simulink model "BEML_EMU_TestBench_6Car"  (R2019b)
settings: Solver=VariableStepAuto  StartTime=0.0  StopTime=inf  RelTol=1e-3
PreLoadFcn:
  | set_up_test_modelCB_6Car;
undefined symbols (not defined in the file): Common, IOControls, MaxVehicles, MotionBaseControllerInput, VehicleInputs, VehicleType, Z_CfgVehBus
libraries: TestBenchLib x583, simulink x6
(part 1 of 3)
settings Model: EnablePacing=on  Creator=bnadpurohit  LastModifiedBy=hinganes
settings DebuggingCC: FrameProcessingCompatibilityMsg=warning

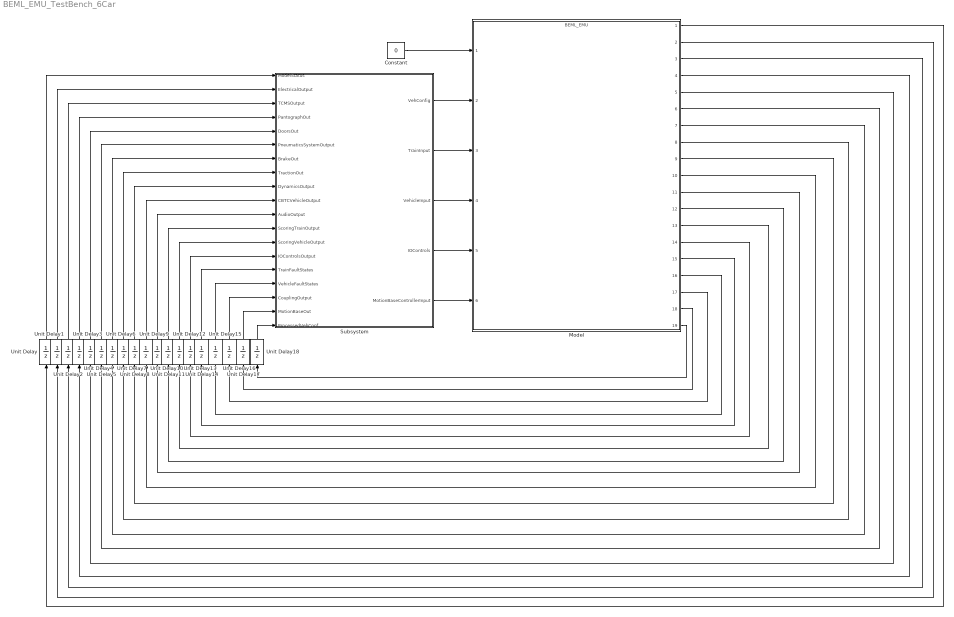
== system BEML_EMU_TestBench_6Car ==
  Constant : Constant  Value=0  OutDataTypeStr=Bus: BD_CommonTrain_SimulatorData
  Model : ModelReference  ModelNameDialog=BEML_EMU.slx  ParameterArgumentNames=PRM_SimIntegration  ParameterArgumentValues=Z_SimIntegrationPrm  UsingDefaultArgumentValue=0  SimulationMode=Normal  ModelReferenceVersion=1.1242
  Subsystem : Subsystem  TreatAsAtomicUnit=on  SystemSampleTime=0.05
  Unit Delay{,1..18} (19 alike) : UnitDelay  SampleTime=-1  HasFrameUpgradeWarning=on
  wires:
  Model/13 -> Unit Delay12/1
  Model/18 -> Unit Delay17/1
  Unit Delay17/1 -> Subsystem/18(MotionBaseOut)
  Model/1 -> Unit Delay/1
  Model/5 -> Unit Delay4/1
  Subsystem/1(VehConfig) -> Model/2
  Model/10 -> Unit Delay9/1
  Model/6 -> Unit Delay5/1
  Unit Delay18/1 -> Subsystem/19(ProcessedVehConf)
  Model/19 -> Unit Delay18/1
  Model/15 -> Unit Delay14/1
  Unit Delay10/1 -> Subsystem/11(AudioOutput)
  Unit Delay6/1 -> Subsystem/7(BrakeOut)
  Subsystem/2(TrainInput) -> Model/3
  Subsystem/5(MotionBaseControllerInput) -> Model/6
  Unit Delay12/1 -> Subsystem/13(ScoringVehicleOutput)
  Unit Delay14/1 -> Subsystem/15(TrainFaultStates)
  Unit Delay2/1 -> Subsystem/3(TCMSOutput)
  Subsystem/3(VehicleInput) -> Model/4
  Unit Delay8/1 -> Subsystem/9(DynamicsOutput)
  Unit Delay11/1 -> Subsystem/12(ScoringTrainOutput)
  Model/4 -> Unit Delay3/1
  Model/2 -> Unit Delay1/1
  Unit Delay1/1 -> Subsystem/2(ElectricalOutput)
  Constant/1 -> Model/1
  Model/12 -> Unit Delay11/1
  Unit Delay4/1 -> Subsystem/5(DoorsOut)
  Unit Delay/1 -> Subsystem/1(ModelStatus)
  Unit Delay15/1 -> Subsystem/16(VehicleFaultStates)
  Model/3 -> Unit Delay2/1
  Unit Delay5/1 -> Subsystem/6(PneumaticsSystemOutput)
  Model/9 -> Unit Delay8/1
  Model/11 -> Unit Delay10/1
  Model/16 -> Unit Delay15/1
  Unit Delay3/1 -> Subsystem/4(PantographOut)
  Model/7 -> Unit Delay6/1
  Model/8 -> Unit Delay7/1
  Subsystem/4(IOControls) -> Model/5
  Unit Delay9/1 -> Subsystem/10(CBTCVehicleOutput)
  Unit Delay13/1 -> Subsystem/14(IOControlsOutput)
  Unit Delay7/1 -> Subsystem/8(TractionOut)
  Model/17 -> Unit Delay16/1
  Unit Delay16/1 -> Subsystem/17(CouplingOutput)
  Model/14 -> Unit Delay13/1

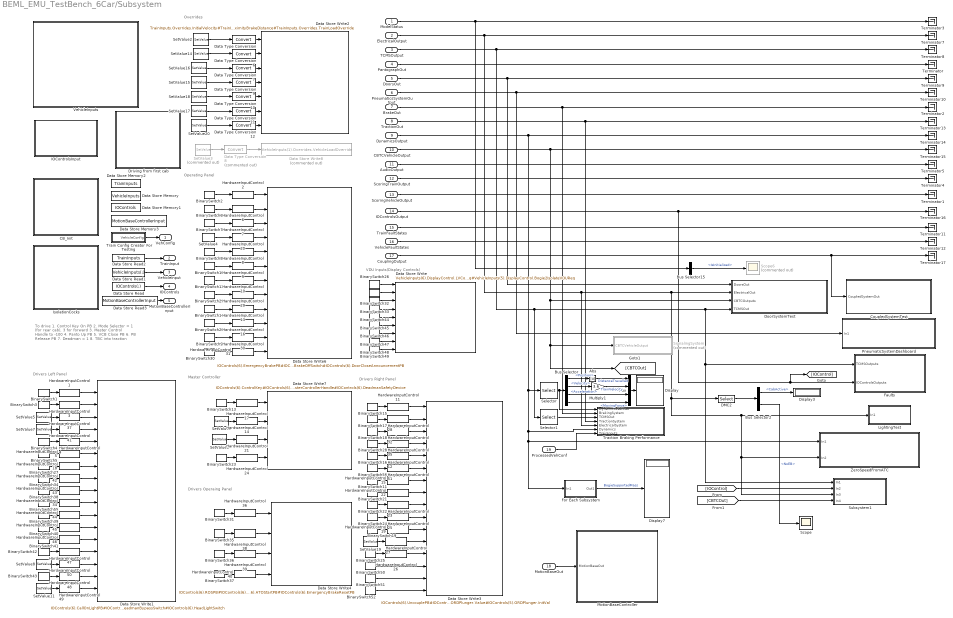
== system BEML_EMU_TestBench_6Car/Subsystem ==
  note: Operating Panel
  note: To drive
      | 1. Control Key On PB
      | 2. Mode Selector = 1 (for rear cab), 3 for forward
      | 3. Master Control Handle to -100
      | 4. Panto Up PB
      | 5. VCB Close PB
      | 6. PB Release PB
      | 7. Deadman = 1
      | 8. TBC into traction
  note: Drivers Operaing Panel
  note: Master Controller
  note: Drivers Right Panel
  note: Drivers Left Panel
  note: VDU Inputs(Display Controls)
  note: Overrides
  ModelStatus : Inport
  ElectricalOutput : Inport  Port=2
  TCMSOutput : Inport  Port=3
  PantographOut : Inport  Port=4
  DoorsOut : Inport  Port=5
  PneumaticsSystemOutput : Inport  Port=6
  BrakeOut : Inport  Port=7
  TractionOut : Inport  Port=8
  DynamicsOutput : Inport  Port=9
  CBTCVehicleOutput : Inport  Port=10
  AudioOutput : Inport  Port=11
  ScoringTrainOutput : Inport  Port=12
  ScoringVehicleOutput : Inport  Port=13
  IOControlsOutput : Inport  Port=14
  TrainFaultStates : Inport  Port=15
  VehicleFaultStates : Inport  Port=16
  CouplingOutput : Inport  Port=17
  MotionBaseOut : Inport  Port=18
  ProcessedVehConf : Inport  Port=19
  Abs : Abs
  BinarySwitch{1..22,24..49,51..52,55..56} (52 alike) : TestBenchLib/BinarySwitch  value=0  init_value=0  block_colour=[0 1 0]  WorkspaceVarName=0
      settings: SourceProductName=Sydac Utilities
  BinarySwitch23 : TestBenchLib/BinarySwitch  value=1  init_value=1  block_colour=[0 1 0]  WorkspaceVarName=0
      settings: SourceProductName=Sydac Utilities
  BinarySwitch50 : TestBenchLib/BinarySwitch  value=1  init_value=1  block_colour=[0 1 0]  WorkspaceVarName=0
      settings: SourceProductName=Sydac Utilities
  Bus Selector : BusSelector  OutputSignals=Inertia.Position,Inertia.Velocity,Inertia.Acceleration,Inertia.MovingForce
  Bus Selector15 : BusSelector  OutputSignals=IsInitialized
  Bus Selector2 : BusSelector  OutputSignals=TCMS.CabActive,TCMS.NoEB
  CB_Init : Subsystem
  CoupledSystemTest : Subsystem
  DMC2 : Selector  InputPortWidth=MaxVehicles  IndexOptions=Index vector (dialog)  Indices=6  OutputSizes=1
  Data Store Memory : DataStoreMemory  DataStoreName=VehicleInputs  ReadBeforeWriteMsg=warning  WriteAfterWriteMsg=warning  WriteAfterReadMsg=warning  ShowAdditionalParam=off  OutDataTypeStr=Bus: BD_SimIntegration_In_Vehicle  Dimensions=MaxVehicles
  Data Store Memory1 : DataStoreMemory  Priority=1  DataStoreName=IOControls  ReadBeforeWriteMsg=warning  WriteAfterWriteMsg=warning  WriteAfterReadMsg=warning  ShowAdditionalParam=off  OutDataTypeStr=Bus: BD_IOControls_In_Vehicle  Dimensions=MaxVehicles
  Data Store Memory2 : DataStoreMemory  DataStoreName=TrainInputs  ReadBeforeWriteMsg=warning  WriteAfterWriteMsg=warning  WriteAfterReadMsg=warning  ShowAdditionalParam=off  OutDataTypeStr=Bus: BD_SimIntegration_In_Train
  Data Store Memory3 : DataStoreMemory  Priority=1  DataStoreName=MotionBaseControllerInput  ReadBeforeWriteMsg=warning  WriteAfterWriteMsg=warning  WriteAfterReadMsg=warning  ShowAdditionalParam=off  OutDataTypeStr=Bus: BD_SimIntegration_In_Vehicle_MotionBaseController  Dimensions=MaxVehicles
  Data Store Read : DataStoreRead  Priority=2  DataStoreName=IOControls  DataStoreElements=IOControls(:)
  Data Store Read1 : DataStoreRead  Priority=2  DataStoreName=VehicleInputs  DataStoreElements=VehicleInputs(:)
  Data Store Read2 : DataStoreRead  Priority=2  DataStoreName=TrainInputs  DataStoreElements=TrainInputs
  Data Store Read3 : DataStoreRead  Priority=2  DataStoreName=MotionBaseControllerInput  DataStoreElements=MotionBaseControllerInput
  Data Store Write : DataStoreWrite  DataStoreName=VehicleInputs  DataStoreElements=VehicleInputs(6).DisplayControl.LVCommandPOPB#VehicleInputs(3).DisplayControl.LVIsolateBCG1#VehicleInputs(3).DisplayControl.LVIsolateBCG2#VehicleInputs(4).DisplayControl.LVIsolateBCG1#VehicleInputs(4).DisplayControl.LVIsolateBCG2#VehicleInputs(6).DisplayControl.Bogie1IsolateVDUReq#VehicleInputs(6).DisplayControl.Bogie2IsolateVDUReq#VehicleInputs(5).DisplayControl.Bogie1IsolateVDUReq#VehicleInputs(5).DisplayControl.Bogie2IsolateVDUReq
  Data Store Write1 : DataStoreWrite  Priority=1  DataStoreName=IOControls  DataStoreElements=IOControls(6).CallOnLightPB#IOControls(6).VCBOpenPB#IOControls(6).WiperSelectionSwitch#IOControls(6).WiperControlSwitch#IOControls(6).LIMPHomePB#IOControls(6).PowerOffPB#IOControls(6).PantoDownPB#IOControls(6).VCBClosePB#IOControls(6).LeftDoorOpenPBOperatingPanel2#IOControls(6).LeftDoorOpenPB1OperatingPanel2#IOControls(6).LeftDoorClosePBOperatingPanel2#IOControls(6).PantoUpPB#IOControls(6).SafetyCutoutSS#IOControls(6).BrakeLoopCutoutSS#IOControls(6).PantoSelector#IOControls(6).DeadmanBypassSwitch#IOControls(6).HeadLightSwitch
  Data Store Write2 : DataStoreWrite  Priority=1  DataStoreName=TrainInputs  DataStoreElements=TrainInputs.Overrides.InitialVelocity#TrainInputs.CBTCTuning.ATOTractionP#TrainInputs.CBTCTuning.ATOTractionI#TrainInputs.CBTCTuning.ATOBrakeP#TrainInputs.CBTCTuning.ATOBrakeI#TrainInputs.CBTCTuning.ATOProximityBrakeDistance#TrainInputs.Overrides.TrainLoadOverride
  Data Store Write3 : DataStoreWrite  Priority=1  DataStoreName=IOControls  DataStoreElements=IOControls(6).UncouplePB#IOControls(6).FlasherLightPB#IOControls(6).FloodLightPB#IOControls(6).BatteryResetPB#IOControls(6).RightDoorOpenPBOperatingPanel5#IOControls(6).RightDoorOpenPB1OperatingPanel5#IOControls(6).RightDoorClosePBOperatingPanel5#IOControls(6).DoorProvenLoopOutputSwitch#IOControls(6).LampTestPB#IOControls(6).WFLTestPB#IOControls(6).EmergencyStopPB#IOControls(6).HoldDoorCloseBypassSS#IOControls(6).EmergencyBrakePBBypassSS#IOControls(5).ORDPlunger.Mode#IOControls(5).ORDPlunger.Value#IOControls(5).ORDPlunger.InitVal
  Data Store Write4 : DataStoreWrite  Priority=1  DataStoreName=IOControls  DataStoreElements=IOControls(6).ROSPB#IOControls(6).UTOPB#IOControls(6).ATOStartPB#IOControls(6).EmergencyBrakeResetPB
  Data Store Write6 : DataStoreWrite  Priority=1  DataStoreName=IOControls  DataStoreElements=IOControls(6).EmergencyBrakePB#IOControls(6).HornPB#IOControls(6).CabConsoleLightPB#IOControls(6).DoorProvenLoopCutoutPB#IOControls(6).LeftDoorClosePBOperatingPanel1#IOControls(6).RightDoorClosePBOperatingPanel1#IOControls(6).LeftDoorOpenPBOperatingPanel1#IOControls(6).RightDoorOpenPBOperatingPanel1#IOControls(6).CabMainLightPB#IOControls(6).ParkingBrakeOnSwitch#IOControls(6).ParkingBrakeOffSwitch#IOControls(6).DoorCloseAnnouncementPB
  Data Store Write7 : DataStoreWrite  Priority=1  DataStoreName=IOControls  DataStoreElements=IOControls(6).ControlKey#IOControls(6).ModeSelector#IOControls(6).MasterControllerHandle#IOControls(6).DeadmanSafetyDevice
  Data Store Write8 : DataStoreWrite  Priority=1  Commented=on  DataStoreName=VehicleInputs  DataStoreElements=VehicleInputs(1).Overrides.VehicleLoadOverride
  Data Type Conversion{,6..7,9..12} (7 alike) : DataTypeConversion
  Data Type Conversion8 : DataTypeConversion  Commented=on
  Display : Display
  Display3 : Display
  Display7 : Display
  DoorSystemTest : Subsystem
  Driving from first cab : Subsystem
  Faults : Subsystem
  For Each Subsystem : Subsystem  TreatAsAtomicUnit=on
  HardwareInputControl{1..32,34..51} (50 alike) : TestBenchLib/HardwareInputControl
      settings: SourceProductName=Sydac Utilities
  IOControlsInput : Subsystem
  IsolationCocks : Subsystem
  LightingTest : Subsystem
  MotionBaseController : Subsystem
  Multiply1 : Gain  Gain=3.6
  Mux : Mux
  PneumaticSystemDashboard : Subsystem
  Scope : Scope
  Scope6 : Scope  Commented=on
  Selector : Selector  InputPortWidth=MaxVehicles  IndexOptions=Index vector (dialog)  Indices=6  OutputSizes=1
  Selector1 : Selector  InputPortWidth=MaxVehicles  IndexOptions=Index vector (dialog)  Indices=6  OutputSizes=1
  SetValue1 : TestBenchLib/SetValue  value=-100  init_value=-100  WorkspaceVarName=0
      settings: SourceProductName=Sydac Utilities
  SetValue{2,4..8,11,19..20} (9 alike) : TestBenchLib/SetValue  value=0  init_value=0  WorkspaceVarName=0
      settings: SourceProductName=Sydac Utilities
  SetValue14 : TestBenchLib/SetValue  value=50  init_value=50  WorkspaceVarName=0
      settings: SourceProductName=Sydac Utilities
  SetValue15 : TestBenchLib/SetValue  value=100  init_value=100  WorkspaceVarName=0
      settings: SourceProductName=Sydac Utilities
  SetValue16 : TestBenchLib/SetValue  value=2  init_value=2  WorkspaceVarName=0
      settings: SourceProductName=Sydac Utilities
  SetValue17 : TestBenchLib/SetValue  value=0.5  init_value=0.5  WorkspaceVarName=0
      settings: SourceProductName=Sydac Utilities
  SetValue18 : TestBenchLib/SetValue  value=5  init_value=5  WorkspaceVarName=0
      settings: SourceProductName=Sydac Utilities
  SetValue3 : TestBenchLib/SetValue  Commented=on  value=0  init_value=0  WorkspaceVarName=0
      settings: SourceProductName=Sydac Utilities
  SignalingSystem : Subsystem  Commented=on
  Subsystem1 : Subsystem
  Terminator{,1..5,7..17} (17 alike) : Terminator
  Traction Braking Performance : Subsystem
  Train Config Creator For Testing : Subsystem
  VehicleInputs : Subsystem
  ZeroSpeedFromATC : Subsystem
  VehConfig : Outport  VectorParamsAs1DForOutWhenUnconnected=off
  TrainInput : Outport  Port=2  VectorParamsAs1DForOutWhenUnconnected=off
  VehicleInput : Outport  Port=3  VectorParamsAs1DForOutWhenUnconnected=off
  IOControls : Outport  Port=4  VectorParamsAs1DForOutWhenUnconnected=off
  MotionBaseControllerInput : Outport  Port=5  VectorParamsAs1DForOutWhenUnconnected=off
  wires:
  BinarySwitch32/1 -> Data Store Write/2
  HardwareInputControl44/1 -> Data Store Write1/11
  BinarySwitch29/1 -> HardwareInputControl29/1
  Selector1/1 -> Traction Braking Performance/3(TCMSOut)
  SetValue4/1 -> HardwareInputControl20/1
  BinarySwitch1/1 -> HardwareInputControl1/1
  SetValue2/1 -> Data Type Conversion/1
  BinarySwitch17/1 -> HardwareInputControl28/1
  BinarySwitch33/1 -> Data Store Write/3
  BinarySwitch13/1 -> HardwareInputControl17/1
  Bus Selector15/1 -> Scope6/1  "<IsInitialized>"
  BinarySwitch56/1 -> HardwareInputControl51/1
  SetValue17/1 -> Data Type Conversion11/1
  Data Type Conversion6/1 -> Data Store Write2/2
  BinarySwitch45/1 -> Data Store Write/5
  Data Type Conversion/1 -> Data Store Write2/1
  SetValue18/1 -> Data Type Conversion10/1
  Data Type Conversion8/1 -> Data Store Write8/1
  HardwareInputControl42/1 -> Data Store Write1/8
  SetValue16/1 -> Data Type Conversion7/1
  Data Type Conversion7/1 -> Data Store Write2/3
  SetValue15/1 -> Data Type Conversion9/1
  HardwareInputControl25/1 -> Data Store Write3/10
  BinarySwitch30/1 -> HardwareInputControl31/1
  Data Type Conversion9/1 -> Data Store Write2/4
  Data Type Conversion10/1 -> Data Store Write2/5
  BinarySwitch12/1 -> HardwareInputControl10/1
  Bus Selector/4 -> Mux/4  "<MovingForce>"
  SetValue5/1 -> HardwareInputControl37/1
  BinarySwitch49/1 -> Data Store Write/9
  BinarySwitch44/1 -> Data Store Write/4
  DMC2/1 -> Bus Selector2/1
  TrainFaultStates/1 -> Terminator11/1
  BinarySwitch47/1 -> Data Store Write/7
  For Each Subsystem/1(Out1) -> Display7/1  "BogieSupportedMass"
  BinarySwitch26/1 -> Data Store Write/1
  HardwareInputControl16/1 -> Data Store Write6/10
  Data Store Read2/1 -> TrainInput/1
  BinarySwitch48/1 -> Data Store Write/8
  HardwareInputControl45/1 -> Data Store Write1/12
  SetValue1/1 -> HardwareInputControl21/1
  Data Type Conversion11/1 -> Data Store Write2/6
  BinarySwitch7/1 -> HardwareInputControl7/1
  SetValue14/1 -> Data Type Conversion6/1
  Mux/1 -> Display/1
  CouplingOutput/1 -> Terminator17/1, CoupledSystemTest/1(CoupledSystemOut)
  Data Type Conversion12/1 -> Data Store Write2/7
  ElectricalOutput/1 -> Terminator7/1, Traction Braking Performance/5(ElectricalSystem), ZeroSpeedFromATC/2(In2), Subsystem1/3(In3), LightingTest/1(In1), DMC2/1, DoorSystemTest/2(ElectricalOut)
  HardwareInputControl2/1 -> Data Store Write6/1
  SetValue3/1 -> Data Type Conversion8/1
  SetValue20/1 -> Data Type Conversion12/1
  HardwareInputControl19/1 -> Data Store Write3/11
  BinarySwitch39/1 -> HardwareInputControl44/1
  CBTCVehicleOutput/1 -> Terminator15/1, DoorSystemTest/3(CBTCOutputs), [CBTCOut], SignalingSystem/1(CBTCVehicleOutput)
  PneumaticsSystemOutput/1 -> Terminator10/1, PneumaticSystemDashboard/1(In1)
  BinarySwitch18/1 -> HardwareInputControl32/1
  HardwareInputControl47/1 -> Data Store Write1/14
  HardwareInputControl11/1 -> Data Store Write3/1
  HardwareInputControl41/1 -> Data Store Write1/4
  BinarySwitch42/1 -> HardwareInputControl47/1
  HardwareInputControl38/1 -> Data Store Write4/2
  Abs/1 -> Mux/1  "DistanceTravelled"
  HardwareInputControl30/1 -> Data Store Write6/11
  HardwareInputControl6/1 -> Data Store Write6/2
  HardwareInputControl26/1 -> Data Store Write3/13
  BinarySwitch36/1 -> HardwareInputControl39/1
  HardwareInputControl50/1 -> Data Store Write1/15
  HardwareInputControl23/1 -> Data Store Write3/9
  HardwareInputControl15/1 -> Data Store Write3/7
  TCMSOutput/1 -> Terminator8/1, Selector1/1, Subsystem1/1(In1), Faults/1(TCMSOutputs), DoorSystemTest/4(TCMSOut)
  HardwareInputControl27/1 -> Data Store Write3/12
  [IOControl] -> Subsystem1/2(In2)
  IOControlsOutput/1 -> Terminator16/1, [IOControl], Faults/2(IOControlsOutputs)
  HardwareInputControl51/1 -> Data Store Write3/6
  HardwareInputControl4/1 -> Data Store Write1/5
  SetValue8/1 -> HardwareInputControl50/1
  Data Store Read1/1 -> VehicleInput/1
  HardwareInputControl3/1 -> Data Store Write1/2
  HardwareInputControl22/1 -> Data Store Write3/8
  [CBTCOut] -> Subsystem1/4(In4)
  HardwareInputControl34/1 -> Data Store Write1/10
  HardwareInputControl46/1 -> Data Store Write1/13
  HardwareInputControl49/1 -> Data Store Write1/17
  BinarySwitch22/1 -> HardwareInputControl23/1
  BinarySwitch55/1 -> HardwareInputControl34/1
  HardwareInputControl28/1 -> Data Store Write3/2
  HardwareInputControl48/1 -> Data Store Write1/16
  BinarySwitch2/1 -> HardwareInputControl2/1
  TractionOut/1 -> Traction Braking Performance/4(TractionSystem), Terminator13/1
  PantographOut/1 -> Terminator/1
  BrakeOut/1 -> Traction Braking Performance/2(BrakingSystem), Terminator2/1
  HardwareInputControl29/1 -> Data Store Write6/8
  ScoringVehicleOutput/1 -> Terminator1/1
  HardwareInputControl8/1 -> Data Store Write6/5
  DoorsOut/1 -> Terminator9/1, DoorSystemTest/1(DoorsOut)
  BinarySwitch37/1 -> HardwareInputControl40/1
  Selector/1 -> Traction Braking Performance/1(DynamicsLastCab), Bus Selector/1
  BinarySwitch27/1 -> HardwareInputControl18/1
  BinarySwitch10/1 -> HardwareInputControl9/1
  SetValue11/1 -> HardwareInputControl49/1
  BinarySwitch24/1 -> HardwareInputControl25/1
  HardwareInputControl21/1 -> Data Store Write7/3
  Train Config Creator For Testing/1(VehicleConfig) -> VehConfig/1
  HardwareInputControl5/1 -> Data Store Write1/6
  HardwareInputControl7/1 -> Data Store Write6/3
  BinarySwitch4/1 -> HardwareInputControl4/1
  Bus Selector/2 -> Multiply1/1  "<Velocity>"
  Multiply1/1 -> Mux/2  "TrainVelocity"
  BinarySwitch5/1 -> HardwareInputControl5/1
  HardwareInputControl1/1 -> Data Store Write1/1
  Bus Selector/3 -> Mux/3  "<Acceleration>"
  HardwareInputControl17/1 -> Data Store Write7/1
  BinarySwitch8/1 -> HardwareInputControl8/1
  HardwareInputControl24/1 -> Data Store Write7/4
  HardwareInputControl12/1 -> Data Store Write3/5
  Bus Selector/1 -> Abs/1  "<Position>"
  HardwareInputControl13/1 -> Data Store Write6/9
  SetValue19/1 -> HardwareInputControl27/1
  BinarySwitch41/1 -> HardwareInputControl46/1
  DynamicsOutput/1 -> Terminator14/1, Traction Braking Performance/6(Dynamics), For Each Subsystem/1(In1), ZeroSpeedFromATC/1(In1), Selector/1
  ModelStatus/1 -> Terminator3/1, Bus Selector15/1
  HardwareInputControl9/1 -> Data Store Write6/6
  BinarySwitch35/1 -> HardwareInputControl38/1
  SetValue6/1 -> HardwareInputControl14/1
  VehicleFaultStates/1 -> Terminator12/1
  BinarySwitch23/1 -> HardwareInputControl24/1
  BinarySwitch14/1 -> HardwareInputControl13/1
  HardwareInputControl35/1 -> Data Store Write3/4
  BinarySwitch19/1 -> HardwareInputControl19/1
  HardwareInputControl14/1 -> Data Store Write7/2
  HardwareInputControl36/1 -> Data Store Write4/1
  SetValue7/1 -> HardwareInputControl41/1
  BinarySwitch6/1 -> HardwareInputControl6/1
  HardwareInputControl18/1 -> Data Store Write1/7
  BinarySwitch28/1 -> HardwareInputControl35/1
  BinarySwitch43/1 -> HardwareInputControl48/1
  HardwareInputControl31/1 -> Data Store Write6/12
  BinarySwitch40/1 -> HardwareInputControl45/1
  BinarySwitch34/1 -> HardwareInputControl42/1
  Bus Selector2/1 -> Display3/1  "<CabActive>"
  BinarySwitch38/1 -> HardwareInputControl43/1
  BinarySwitch15/1 -> HardwareInputControl11/1
  Data Store Read/1 -> IOControls/1
  HardwareInputControl43/1 -> Data Store Write1/9
  BinarySwitch3/1 -> HardwareInputControl3/1
  AudioOutput/1 -> Terminator5/1
  HardwareInputControl10/1 -> Data Store Write6/7
  BinarySwitch25/1 -> HardwareInputControl26/1
  BinarySwitch21/1 -> HardwareInputControl22/1
  ScoringTrainOutput/1 -> Terminator4/1
  HardwareInputControl39/1 -> Data Store Write4/3
  HardwareInputControl37/1 -> Data Store Write1/3
  BinarySwitch11/1 -> HardwareInputControl15/1
  BinarySwitch31/1 -> HardwareInputControl36/1
  HardwareInputControl32/1 -> Data Store Write3/3
  BinarySwitch46/1 -> Data Store Write/6
  BinarySwitch9/1 -> HardwareInputControl30/1
  BinarySwitch20/1 -> HardwareInputControl16/1
  HardwareInputControl20/1 -> Data Store Write6/4
  BinarySwitch16/1 -> HardwareInputControl12/1
  HardwareInputControl40/1 -> Data Store Write4/4
  Bus Selector2/2 -> Scope/1  "<NoEB>"
  Data Store Read3/1 -> MotionBaseControllerInput/1
  MotionBaseOut/1 -> MotionBaseController/1(MotionBaseOut)
  ProcessedVehConf/1 -> Traction Braking Performance/7(TrainInputs)
  BinarySwitch50/1 -> Data Store Write3/14
  BinarySwitch51/1 -> Data Store Write3/15
  BinarySwitch52/1 -> Data Store Write3/16

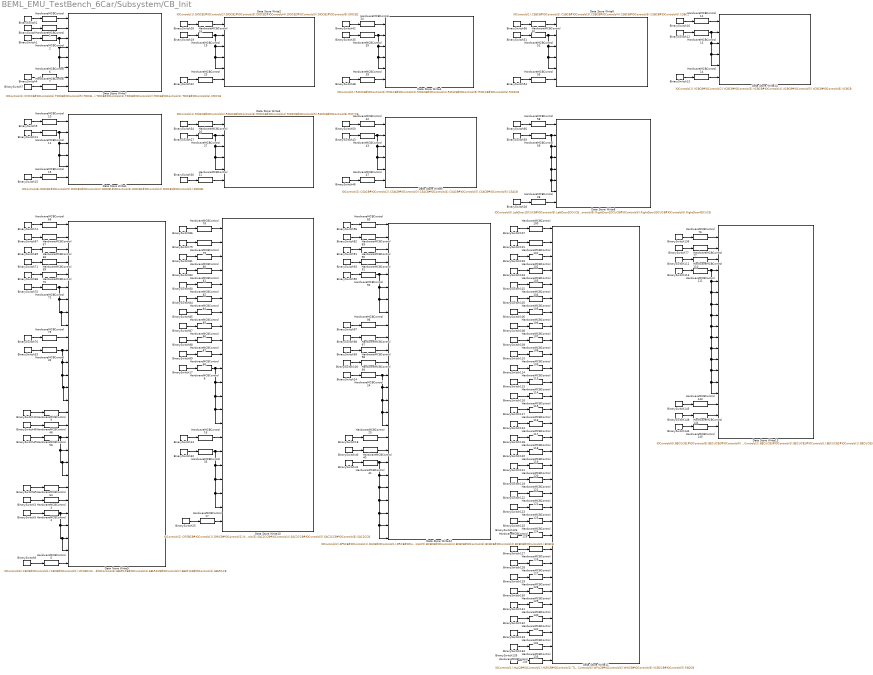
== system BEML_EMU_TestBench_6Car/Subsystem/CB_Init ==
  BinarySwitch{1..19,22,24..28,30,32..35,38,40..43,46,48..51,54,58..59,65..71,74,76..77,79..91,93,96..111,113..136,144..145,148} (110 alike) : TestBenchLib/BinarySwitch  value=1  init_value=1  block_colour=[0 1 0]  WorkspaceVarName=0
      settings: SourceProductName=Sydac Utilities
  Data Store Write1 : DataStoreWrite  Priority=1  DataStoreName=IOControls  DataStoreElements=IOControls(6).DIOCB1#IOControls(5).DIOCB1#IOControls(4).DIOCB1#IOControls(3).DIOCB1#IOControls(2).DIOCB1#IOControls(1).DIOCB1
  Data Store Write10 : DataStoreWrite  Priority=1  DataStoreName=IOControls  DataStoreElements=IOControls(1).CRSBCB#IOControls(1).DMICB#IOControls(1).NVICB#IOControls(1).VIO1CB#IOControls(1).VIO2CB#IOControls(6).CRSBCB#IOControls(6).DMICB#IOControls(6).NVICB#IOControls(6).VIO1CB#IOControls(6).VIO2CB#IOControls(1).SAC1CCB#IOControls(2).SAC1CCB#IOControls(3).SAC1CCB#IOControls(4).SAC1CCB#IOControls(5).SAC1CCB#IOControls(6).SAC1CCB#IOControls(1).SAC2CCB#IOControls(2).SAC2CCB#IOControls(3).SAC2CCB#IOControls(4).SAC2CCB#IOControls(5).SAC2CCB#IOControls(6).SAC2CCB
  Data Store Write11 : DataStoreWrite  Priority=1  DataStoreName=IOControls  DataStoreElements=IOControls(1).HLLCB#IOControls(1).HLRCB#IOControls(1).TLLCB#IOControls(1).TLRCB#IOControls(1).CELCB#IOControls(1).ILCB1#IOControls(1).ILCB2#IOControls(1).TBCCB1#IOControls(1).TBCCB2#IOControls(1).POCB#IOControls(1).ODDCB#IOControls(1).WFLCB#IOControls(1).WWCB#IOControls(1).VCBCCB#IOControls(2).PADCB#IOControls(2).PANCB#IOControls(5).PANCB#IOControls(6).HLLCB#IOControls(6).HLRCB#IOControls(6).TLLCB#IOControls(6).TLRCB#IOControls(6).CELCB#IOControls(6).ILCB1#IOControls(6).ILCB2#IOControls(6).TBCCB1#IOControls(6).TBCCB2#IOControls(6).POCB#IOControls(6).ODDCB#IOControls(6).WFLCB#IOControls(6).WWCB#IOControls(6).VCBCCB#IOControls(5).PADCB
  Data Store Write12 : DataStoreWrite  Priority=1  DataStoreName=IOControls  DataStoreElements=IOControls(2).APSCB#IOControls(1).DLCB#IOControls(1).DRCB#IOControls(6).DPLCB#IOControls(5).DPLCB#IOControls(4).DPLCB#IOControls(3).DPLCB#IOControls(2).DPLCB#IOControls(1).DPLCB#IOControls(5).APSCB#IOControls(6).DLCB#IOControls(6).DRCB#IOControls(1).AC1CB#IOControls(2).AC1CB#IOControls(3).AC1CB#IOControls(4).AC1CB#IOControls(5).AC1CB#IOControls(6).AC1CB#IOControls(6).EDCB#IOControls(1).EDCB#IOControls(6).BCBCB#IOControls(5).BCBCB#IOControls(4).BCBCB#IOControls(3).BCBCB#IOControls(2).BCBCB#IOControls(1).BCBCB
  Data Store Write13 : DataStoreWrite  Priority=1  DataStoreName=IOControls  DataStoreElements=IOControls(6).BECUCB1#IOControls(6).BECUCB2#IOControls(6).BECUCB3#IOControls(5).BECUCB1#IOControls(5).BECUCB2#IOControls(5).BECUCB3#IOControls(4).BECUCB1#IOControls(4).BECUCB2#IOControls(4).BECUCB3#IOControls(3).BECUCB1#IOControls(3).BECUCB2#IOControls(3).BECUCB3#IOControls(2).BECUCB1#IOControls(2).BECUCB2#IOControls(2).BECUCB3#IOControls(1).BECUCB1#IOControls(1).BECUCB2#IOControls(1).BECUCB3
  Data Store Write14 : DataStoreWrite  Priority=1  DataStoreName=IOControls  DataStoreElements=IOControls(1).VCBCB#IOControls(2).VCBCB#IOControls(3).VCBCB#IOControls(4).VCBCB#IOControls(5).VCBCB#IOControls(6).VCBCB
  Data Store Write2 : DataStoreWrite  Priority=1  DataStoreName=IOControls  DataStoreElements=IOControls(1).DIOCB2#IOControls(2).DIOCB2#IOControls(3).DIOCB2#IOControls(4).DIOCB2#IOControls(5).DIOCB2#IOControls(6).DIOCB2
  Data Store Write3 : DataStoreWrite  Priority=1  DataStoreName=IOControls  DataStoreElements=IOControls(1).RIO2CB#IOControls(2).RIO2CB#IOControls(3).RIO2CB#IOControls(4).RIO2CB#IOControls(5).RIO2CB#IOControls(6).RIO2CB
  Data Store Write4 : DataStoreWrite  Priority=1  DataStoreName=IOControls  DataStoreElements=IOControls(1).RIO1CB#IOControls(2).RIO1CB#IOControls(3).RIO1CB#IOControls(4).RIO1CB#IOControls(5).RIO1CB#IOControls(6).RIO1CB
  Data Store Write5 : DataStoreWrite  Priority=1  DataStoreName=IOControls  DataStoreElements=IOControls(1).CSACB#IOControls(2).CSACB#IOControls(3).CSACB#IOControls(4).CSACB#IOControls(5).CSACB#IOControls(6).CSACB
  Data Store Write6 : DataStoreWrite  Priority=1  DataStoreName=IOControls  DataStoreElements=IOControls(1).CSBCB#IOControls(2).CSBCB#IOControls(3).CSBCB#IOControls(4).CSBCB#IOControls(5).CSBCB#IOControls(6).CSBCB
  Data Store Write7 : DataStoreWrite  Priority=1  DataStoreName=IOControls  DataStoreElements=IOControls(1).CMCCB#IOControls(6).TDICB#IOControls(5).TDICB#IOControls(4).TDICB#IOControls(3).TDICB#IOControls(2).TDICB#IOControls(1).TDICB#IOControls(6).CMCCB
  Data Store Write8 : DataStoreWrite  Priority=1  DataStoreName=IOControls  DataStoreElements=IOControls(6).LeftDoor1DCUCB#IOControls(6).LeftDoor2DCUCB#IOControls(6).LeftDoor3DCUCB#IOControls(6).LeftDoor4DCUCB#IOControls(6).RightDoor1DCUCB#IOControls(6).RightDoor2DCUCB#IOControls(6).RightDoor3DCUCB#IOControls(6).RightDoor4DCUCB
  Data Store Write9 : DataStoreWrite  Priority=1  DataStoreName=IOControls  DataStoreElements=IOControls(6).CECB#IOControls(1).CECB#IOControls(1).VCCBOrUCCB#IOControls(6).VCCBOrUCCB#IOControls(6).BLCB#IOControls(5).BLCB#IOControls(4).BLCB#IOControls(3).BLCB#IOControls(2).BLCB#IOControls(1).BLCB#IOControls(6).TVDUCB#IOControls(5).TVDUCB#IOControls(4).TVDUCB#IOControls(3).TVDUCB#IOControls(2).TVDUCB#IOControls(1).TVDUCB#IOControls(6).BCGCB#IOControls(5).BCGCB#IOControls(4).BCGCB#IOControls(3).BCGCB#IOControls(2).BCGCB#IOControls(1).BCGCB#IOControls(6).EBLR1CB#IOControls(5).EBLR1CB#IOControls(4).EBLR1CB#IOControls(3).EBLR1CB#IOControls(2).EBLR1CB#IOControls(1).EBLR1CB
  HardwareMCBControl{,1..19,23..28,31..35,39..43,47..48,50..51,55..56,58..59,64,66..71,75..92,96..111,113..134,143..145} (110 alike) : TestBenchLib/HardwareMCBControl
      settings: SourceProductName=Sydac Utilities
  wires:
  BinarySwitch30/1 -> HardwareMCBControl31/1
  BinarySwitch26/1 -> HardwareMCBControl18/1
  HardwareMCBControl18/1 -> Data Store Write2/1
  BinarySwitch1/1 -> HardwareMCBControl2/1
  HardwareMCBControl11/1 -> Data Store Write1/3, Data Store Write1/4, Data Store Write1/5, Data Store Write1/2
  HardwareMCBControl15/1 -> Data Store Write1/6
  BinarySwitch11/1 -> HardwareMCBControl11/1
  BinarySwitch15/1 -> HardwareMCBControl15/1
  BinarySwitch6/1 -> HardwareMCBControl1/1
  BinarySwitch4/1 -> HardwareMCBControl6/1
  BinarySwitch2/1 -> HardwareMCBControl/1
  BinarySwitch66/1 -> HardwareMCBControl58/1
  BinarySwitch46/1 -> HardwareMCBControl47/1
  HardwareMCBControl35/1 -> Data Store Write4/3, Data Store Write4/4, Data Store Write4/5, Data Store Write4/2
  BinarySwitch22/1 -> HardwareMCBControl23/1
  HardwareMCBControl27/1 -> Data Store Write3/3, Data Store Write3/4, Data Store Write3/5, Data Store Write3/2
  HardwareMCBControl1/1 -> Data Store Write7/2
  HardwareMCBControl39/1 -> Data Store Write4/6
  BinarySwitch43/1 -> HardwareMCBControl43/1
  BinarySwitch7/1 -> HardwareMCBControl7/1
  HardwareMCBControl58/1 -> Data Store Write8/1
  HardwareMCBControl50/1 -> Data Store Write6/1
  BinarySwitch59/1 -> HardwareMCBControl59/1
  BinarySwitch58/1 -> HardwareMCBControl50/1
  HardwareMCBControl55/1 -> Data Store Write6/6
  HardwareMCBControl43/1 -> Data Store Write5/3, Data Store Write5/4, Data Store Write5/5, Data Store Write5/2
  HardwareMCBControl10/1 -> Data Store Write1/1
  HardwareMCBControl23/1 -> Data Store Write2/6
  HardwareMCBControl59/1 -> Data Store Write8/4, Data Store Write8/6, Data Store Write8/7, Data Store Write8/5, Data Store Write8/3, Data Store Write8/2
  BinarySwitch9/1 -> HardwareMCBControl10/1
  HardwareMCBControl34/1 -> Data Store Write4/1
  HardwareMCBControl2/1 -> Data Store Write7/4, Data Store Write7/5, Data Store Write7/6, Data Store Write7/3
  HardwareMCBControl51/1 -> Data Store Write6/3, Data Store Write6/4, Data Store Write6/5, Data Store Write6/2
  BinarySwitch54/1 -> HardwareMCBControl55/1
  BinarySwitch42/1 -> HardwareMCBControl34/1
  HardwareMCBControl7/1 -> Data Store Write7/8
  BinarySwitch38/1 -> HardwareMCBControl39/1
  HardwareMCBControl47/1 -> Data Store Write5/6
  HardwareMCBControl6/1 -> Data Store Write7/7
  BinarySwitch50/1 -> HardwareMCBControl42/1
  HardwareMCBControl42/1 -> Data Store Write5/1
  HardwareMCBControl/1 -> Data Store Write7/1
  BinarySwitch19/1 -> HardwareMCBControl19/1
  BinarySwitch51/1 -> HardwareMCBControl51/1
  HardwareMCBControl26/1 -> Data Store Write3/1
  HardwareMCBControl19/1 -> Data Store Write2/3, Data Store Write2/4, Data Store Write2/5, Data Store Write2/2
  BinarySwitch34/1 -> HardwareMCBControl26/1
  BinarySwitch27/1 -> HardwareMCBControl27/1
  HardwareMCBControl31/1 -> Data Store Write3/6
  BinarySwitch35/1 -> HardwareMCBControl35/1
  HardwareMCBControl69/1 -> Data Store Write9/4
  BinarySwitch74/1 -> HardwareMCBControl66/1
  HardwareMCBControl68/1 -> Data Store Write9/3
  HardwareMCBControl66/1 -> Data Store Write9/1
  HardwareMCBControl70/1 -> Data Store Write9/5
  BinarySwitch69/1 -> HardwareMCBControl68/1
  BinarySwitch70/1 -> HardwareMCBControl71/1
  BinarySwitch67/1 -> HardwareMCBControl67/1
  BinarySwitch71/1 -> HardwareMCBControl69/1
  HardwareMCBControl71/1 -> Data Store Write9/7, Data Store Write9/8, Data Store Write9/9, Data Store Write9/6
  HardwareMCBControl67/1 -> Data Store Write9/2
  BinarySwitch68/1 -> HardwareMCBControl70/1
  HardwareMCBControl75/1 -> Data Store Write9/10
  BinarySwitch76/1 -> HardwareMCBControl75/1
  HardwareMCBControl88/1 -> Data Store Write10/10
  HardwareMCBControl86/1 -> Data Store Write10/8
  BinarySwitch88/1 -> HardwareMCBControl87/1
  HardwareMCBControl87/1 -> Data Store Write10/9
  BinarySwitch89/1 -> HardwareMCBControl88/1
  BinarySwitch87/1 -> HardwareMCBControl86/1
  BinarySwitch85/1 -> HardwareMCBControl85/1
  BinarySwitch80/1 -> HardwareMCBControl82/1
  HardwareMCBControl85/1 -> Data Store Write10/7
  BinarySwitch84/1 -> HardwareMCBControl84/1
  HardwareMCBControl79/1 -> Data Store Write10/2
  BinarySwitch83/1 -> HardwareMCBControl81/1
  BinarySwitch79/1 -> HardwareMCBControl79/1
  BinarySwitch81/1 -> HardwareMCBControl80/1
  HardwareMCBControl82/1 -> Data Store Write10/5
  HardwareMCBControl78/1 -> Data Store Write10/1
  HardwareMCBControl80/1 -> Data Store Write10/3
  BinarySwitch86/1 -> HardwareMCBControl78/1
  HardwareMCBControl84/1 -> Data Store Write10/6
  HardwareMCBControl81/1 -> Data Store Write10/4
  HardwareMCBControl103/1 -> Data Store Write11/4
  HardwareMCBControl105/1 -> Data Store Write11/6
  BinarySwitch107/1 -> HardwareMCBControl100/1
  HardwareMCBControl102/1 -> Data Store Write11/3
  HardwareMCBControl100/1 -> Data Store Write11/1
  HardwareMCBControl104/1 -> Data Store Write11/5
  BinarySwitch103/1 -> HardwareMCBControl102/1
  BinarySwitch101/1 -> HardwareMCBControl101/1
  BinarySwitch104/1 -> HardwareMCBControl103/1
  HardwareMCBControl101/1 -> Data Store Write11/2
  BinarySwitch105/1 -> HardwareMCBControl105/1
  HardwareMCBControl106/1 -> Data Store Write11/7
  BinarySwitch102/1 -> HardwareMCBControl104/1
  BinarySwitch106/1 -> HardwareMCBControl106/1
  BinarySwitch108/1 -> HardwareMCBControl107/1
  BinarySwitch110/1 -> HardwareMCBControl109/1
  HardwareMCBControl108/1 -> Data Store Write11/9
  BinarySwitch109/1 -> HardwareMCBControl108/1
  HardwareMCBControl107/1 -> Data Store Write11/8
  HardwareMCBControl109/1 -> Data Store Write11/10
  HardwareMCBControl98/1 -> Data Store Write12/11
  HardwareMCBControl96/1 -> Data Store Write12/9
  BinarySwitch98/1 -> HardwareMCBControl97/1
  HardwareMCBControl97/1 -> Data Store Write12/10
  BinarySwitch99/1 -> HardwareMCBControl98/1
  HardwareMCBControl99/1 -> Data Store Write12/12
  BinarySwitch97/1 -> HardwareMCBControl96/1
  BinarySwitch100/1 -> HardwareMCBControl99/1
  BinarySwitch90/1 -> HardwareMCBControl92/1
  HardwareMCBControl89/1 -> Data Store Write12/2
  BinarySwitch93/1 -> HardwareMCBControl91/1
  BinarySwitch82/1 -> HardwareMCBControl89/1
  BinarySwitch91/1 -> HardwareMCBControl90/1
  HardwareMCBControl92/1 -> Data Store Write12/6, Data Store Write12/7, Data Store Write12/8, Data Store Write12/5
  HardwareMCBControl83/1 -> Data Store Write12/1
  HardwareMCBControl90/1 -> Data Store Write12/3
  BinarySwitch96/1 -> HardwareMCBControl83/1
  HardwareMCBControl91/1 -> Data Store Write12/4
  HardwareMCBControl116/1 -> Data Store Write11/14
  HardwareMCBControl114/1 -> Data Store Write11/12
  BinarySwitch116/1 -> HardwareMCBControl115/1
  HardwareMCBControl115/1 -> Data Store Write11/13
  BinarySwitch117/1 -> HardwareMCBControl116/1
  BinarySwitch115/1 -> HardwareMCBControl114/1
  BinarySwitch114/1 -> HardwareMCBControl113/1
  HardwareMCBControl113/1 -> Data Store Write11/11
  HardwareMCBControl118/1 -> Data Store Write11/16
  HardwareMCBControl122/1 -> Data Store Write11/20
  BinarySwitch119/1 -> HardwareMCBControl121/1
  HardwareMCBControl121/1 -> Data Store Write11/19
  HardwareMCBControl130/1 -> Data Store Write11/28
  BinarySwitch121/1 -> HardwareMCBControl120/1
  BinarySwitch129/1 -> HardwareMCBControl128/1
  HardwareMCBControl126/1 -> Data Store Write11/24
  HardwareMCBControl125/1 -> Data Store Write11/23
  BinarySwitch127/1 -> HardwareMCBControl126/1
  HardwareMCBControl124/1 -> Data Store Write11/22
  BinarySwitch126/1 -> HardwareMCBControl125/1
  HardwareMCBControl119/1 -> Data Store Write11/17
  HardwareMCBControl123/1 -> Data Store Write11/21
  BinarySwitch120/1 -> HardwareMCBControl119/1
  BinarySwitch123/1 -> HardwareMCBControl123/1
  HardwareMCBControl120/1 -> Data Store Write11/18
  HardwareMCBControl117/1 -> Data Store Write11/15
  BinarySwitch124/1 -> HardwareMCBControl117/1
  BinarySwitch130/1 -> HardwareMCBControl129/1
  BinarySwitch128/1 -> HardwareMCBControl127/1
  BinarySwitch131/1 -> HardwareMCBControl130/1
  BinarySwitch122/1 -> HardwareMCBControl122/1
  BinarySwitch118/1 -> HardwareMCBControl118/1
  HardwareMCBControl128/1 -> Data Store Write11/26
  HardwareMCBControl129/1 -> Data Store Write11/27
  BinarySwitch125/1 -> HardwareMCBControl124/1
  HardwareMCBControl127/1 -> Data Store Write11/25
  BinarySwitch132/1 -> HardwareMCBControl131/1
  BinarySwitch133/1 -> HardwareMCBControl132/1
  BinarySwitch134/1 -> HardwareMCBControl133/1
  HardwareMCBControl134/1 -> Data Store Write11/32
  HardwareMCBControl131/1 -> Data Store Write11/29
  HardwareMCBControl133/1 -> Data Store Write11/31
  BinarySwitch135/1 -> HardwareMCBControl134/1
  HardwareMCBControl132/1 -> Data Store Write11/30
  HardwareMCBControl25/1 -> Data Store Write12/18
  BinarySwitch18/1 -> HardwareMCBControl25/1
  HardwareMCBControl24/1 -> Data Store Write12/16, Data Store Write12/17, Data Store Write12/15, Data Store Write12/14, Data Store Write12/13
  BinarySwitch24/1 -> HardwareMCBControl24/1
  BinarySwitch17/1 -> HardwareMCBControl8/1
  HardwareMCBControl8/1 -> Data Store Write10/12, Data Store Write10/13, Data Store Write10/14, Data Store Write10/15, Data Store Write10/11
  BinarySwitch14/1 -> HardwareMCBControl16/1
  HardwareMCBControl16/1 -> Data Store Write10/16
  HardwareMCBControl17/1 -> Data Store Write10/22
  BinarySwitch25/1 -> HardwareMCBControl17/1
  HardwareMCBControl33/1 -> Data Store Write10/17, Data Store Write10/18, Data Store Write10/19, Data Store Write10/21, Data Store Write10/20
  BinarySwitch32/1 -> HardwareMCBControl33/1
  BinarySwitch33/1 -> HardwareMCBControl32/1
  HardwareMCBControl32/1 -> Data Store Write9/14, Data Store Write9/15, Data Store Write9/13, Data Store Write9/12, Data Store Write9/11
  BinarySwitch10/1 -> HardwareMCBControl9/1
  HardwareMCBControl9/1 -> Data Store Write9/16
  BinarySwitch40/1 -> HardwareMCBControl40/1
  HardwareMCBControl40/1 -> Data Store Write12/19
  BinarySwitch41/1 -> HardwareMCBControl41/1
  HardwareMCBControl41/1 -> Data Store Write12/24, Data Store Write12/25, Data Store Write12/26, Data Store Write12/23, Data Store Write12/22, Data Store Write12/21, Data Store Write12/20
  HardwareMCBControl48/1 -> Data Store Write9/17
  BinarySwitch48/1 -> HardwareMCBControl48/1
  HardwareMCBControl56/1 -> Data Store Write9/19, Data Store Write9/20, Data Store Write9/21, Data Store Write9/18
  BinarySwitch49/1 -> HardwareMCBControl56/1
  HardwareMCBControl64/1 -> Data Store Write9/22
  BinarySwitch65/1 -> HardwareMCBControl64/1
  BinarySwitch136/1 -> HardwareMCBControl76/1
  HardwareMCBControl111/1 -> Data Store Write13/5, Data Store Write13/6, Data Store Write13/7, Data Store Write13/8, Data Store Write13/9, Data Store Write13/10, Data Store Write13/11, Data Store Write13/12, Data Store Write13/13, Data Store Write13/14, Data Store Write13/15, Data Store Write13/4
  BinarySwitch113/1 -> HardwareMCBControl111/1
  HardwareMCBControl110/1 -> Data Store Write13/3
  BinarySwitch77/1 -> HardwareMCBControl77/1
  HardwareMCBControl77/1 -> Data Store Write13/2
  BinarySwitch111/1 -> HardwareMCBControl110/1
  HardwareMCBControl76/1 -> Data Store Write13/1
  BinarySwitch145/1 -> HardwareMCBControl143/1
  BinarySwitch148/1 -> HardwareMCBControl144/1
  BinarySwitch144/1 -> HardwareMCBControl145/1
  HardwareMCBControl143/1 -> Data Store Write13/16
  HardwareMCBControl144/1 -> Data Store Write13/17
  HardwareMCBControl145/1 -> Data Store Write13/18
  BinarySwitch8/1 -> HardwareMCBControl5/1
  HardwareMCBControl5/1 -> Data Store Write9/28
  BinarySwitch5/1 -> HardwareMCBControl4/1
  HardwareMCBControl4/1 -> Data Store Write9/24, Data Store Write9/25, Data Store Write9/26, Data Store Write9/27
  BinarySwitch3/1 -> HardwareMCBControl3/1
  HardwareMCBControl3/1 -> Data Store Write9/23
  BinarySwitch13/1 -> HardwareMCBControl14/1
  HardwareMCBControl13/1 -> Data Store Write14/2, Data Store Write14/5, Data Store Write14/4, Data Store Write14/3
  BinarySwitch16/1 -> HardwareMCBControl12/1
  BinarySwitch12/1 -> HardwareMCBControl13/1
  HardwareMCBControl14/1 -> Data Store Write14/6
  HardwareMCBControl12/1 -> Data Store Write14/1
  HardwareMCBControl28/1 -> Data Store Write8/8
  BinarySwitch28/1 -> HardwareMCBControl28/1

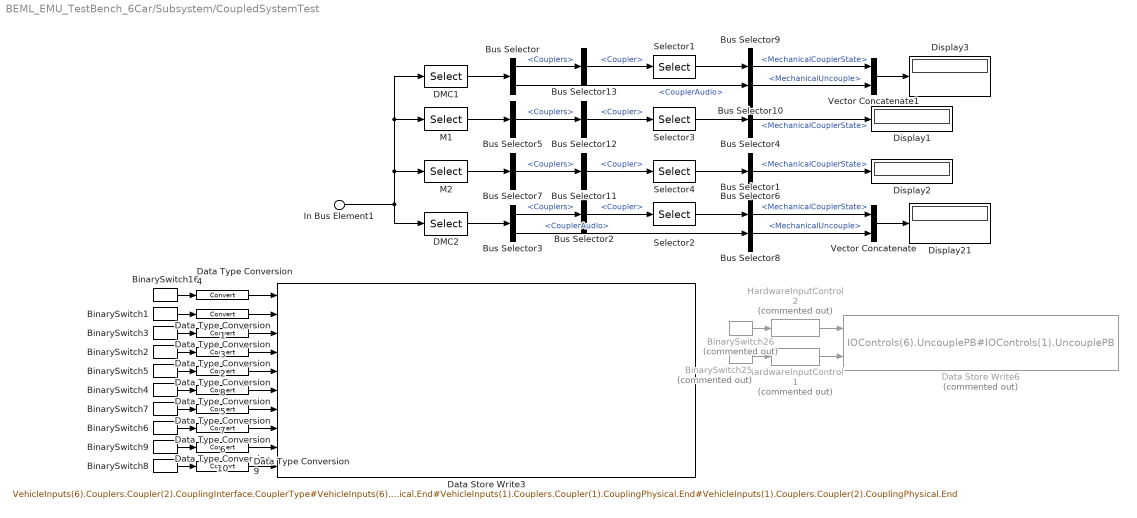
== system BEML_EMU_TestBench_6Car/Subsystem/CoupledSystemTest ==
  In Bus Element1 : Inport  PortName=CoupledSystemOut
  BinarySwitch{1..6,8,16} (8 alike) : TestBenchLib/BinarySwitch  value=0  init_value=0  block_colour=[0 1 0]  WorkspaceVarName=0
      settings: SourceProductName=Sydac Utilities
  BinarySwitch25 : TestBenchLib/BinarySwitch  Commented=on  value=0  init_value=0  block_colour=[0 1 0]  WorkspaceVarName=0
      settings: SourceProductName=Sydac Utilities
  BinarySwitch26 : TestBenchLib/BinarySwitch  Commented=on  value=0  init_value=0  block_colour=[0 1 0]  WorkspaceVarName=0
      settings: SourceProductName=Sydac Utilities
  BinarySwitch7 : TestBenchLib/BinarySwitch  value=1  init_value=1  block_colour=[0 1 0]  WorkspaceVarName=0
      settings: SourceProductName=Sydac Utilities
  BinarySwitch9 : TestBenchLib/BinarySwitch  value=1  init_value=1  block_colour=[0 1 0]  WorkspaceVarName=0
      settings: SourceProductName=Sydac Utilities
  Bus Selector : BusSelector  OutputSignals=Couplers,CouplerAudio
  Bus Selector{1,4,6,9} (4 alike) : BusSelector  OutputSignals=PhysicalSignals.MechanicalCouplerState
  Bus Selector10 : BusSelector  OutputSignals=MechanicalUncouple
  Bus Selector{2,11..13} (4 alike) : BusSelector  OutputSignals=Coupler
  Bus Selector3 : BusSelector  OutputSignals=Couplers,CouplerAudio
  Bus Selector5 : BusSelector  OutputSignals=Couplers
  Bus Selector7 : BusSelector  OutputSignals=Couplers
  Bus Selector8 : BusSelector  OutputSignals=MechanicalUncouple
  DMC1 : Selector  InputPortWidth=MaxVehicles  IndexOptions=Index vector (dialog)  Indices=1  OutputSizes=1
  DMC2 : Selector  InputPortWidth=MaxVehicles  IndexOptions=Index vector (dialog)  Indices=6  OutputSizes=1
  Data Store Write3 : DataStoreWrite  Priority=1  DataStoreName=VehicleInputs  DataStoreElements=VehicleInputs(6).Couplers.Coupler(2).CouplingInterface.CouplerType#VehicleInputs(6).Couplers.Coupler(2).CouplingInterface.ReadyToCouple#VehicleInputs(6).Couplers.Coupler(2).CouplingPhysical.Available#VehicleInputs(1).Couplers.Coupler(1).CouplingInterface.CouplerType#VehicleInputs(1).Couplers.Coupler(1).CouplingInterface.ReadyToCouple#VehicleInputs(1).Couplers.Coupler(1).CouplingPhysical.Available#VehicleInputs(6).Couplers.Coupler(1).CouplingPhysical.End#VehicleInputs(6).Couplers.Coupler(2).CouplingPhysical.End#VehicleInputs(1).Couplers.Coupler(1).CouplingPhysical.End#VehicleInputs(1).Couplers.Coupler(2).CouplingPhysical.End
  Data Store Write6 : DataStoreWrite  Priority=1  Commented=on  DataStoreName=IOControls  DataStoreElements=IOControls(6).UncouplePB#IOControls(1).UncouplePB
  Data Type Conversion{1..10} (10 alike) : DataTypeConversion
  Display{1..3,21} (4 alike) : Display
  HardwareInputControl1 : TestBenchLib/HardwareInputControl  Commented=on
      settings: SourceProductName=Sydac Utilities
  HardwareInputControl2 : TestBenchLib/HardwareInputControl  Commented=on
      settings: SourceProductName=Sydac Utilities
  M1 : Selector  InputPortWidth=MaxVehicles  IndexOptions=Index vector (dialog)  Indices=3  OutputSizes=1
  M2 : Selector  InputPortWidth=MaxVehicles  IndexOptions=Index vector (dialog)  Indices=4  OutputSizes=1
  Selector1 : Selector  InputPortWidth=2  IndexOptions=Index vector (dialog)  Indices=1  OutputSizes=1
  Selector2 : Selector  InputPortWidth=2  IndexOptions=Index vector (dialog)  Indices=2  OutputSizes=1
  Selector3 : Selector  InputPortWidth=2  IndexOptions=Index vector (dialog)  Indices=1  OutputSizes=1
  Selector4 : Selector  InputPortWidth=2  IndexOptions=Index vector (dialog)  Indices=1  OutputSizes=1
  Vector Concatenate : Concatenate
  Vector Concatenate1 : Concatenate
  wires:
  BinarySwitch16/1 -> Data Type Conversion4/1
  Data Type Conversion4/1 -> Data Store Write3/1
  Data Type Conversion1/1 -> Data Store Write3/2
  BinarySwitch1/1 -> Data Type Conversion1/1
  BinarySwitch2/1 -> Data Type Conversion2/1
  Data Type Conversion2/1 -> Data Store Write3/4
  Data Type Conversion3/1 -> Data Store Write3/3
  BinarySwitch3/1 -> Data Type Conversion3/1
  BinarySwitch4/1 -> Data Type Conversion5/1
  Data Type Conversion5/1 -> Data Store Write3/6
  Data Type Conversion8/1 -> Data Store Write3/5
  BinarySwitch5/1 -> Data Type Conversion8/1
  DMC1/1 -> Bus Selector/1
  DMC2/1 -> Bus Selector3/1
  Bus Selector3/1 -> Bus Selector2/1  "<Couplers>"
  Selector2/1 -> Bus Selector1/1
  Selector3/1 -> Bus Selector4/1
  Bus Selector5/1 -> Bus Selector12/1  "<Couplers>"
  M1/1 -> Bus Selector5/1
  Bus Selector4/1 -> Display1/1  "<MechanicalCouplerState>"
  Bus Selector6/1 -> Display2/1  "<MechanicalCouplerState>"
  M2/1 -> Bus Selector7/1
  Bus Selector7/1 -> Bus Selector11/1  "<Couplers>"
  Selector4/1 -> Bus Selector6/1
  In Bus Element1/1 -> M2/1, M1/1, DMC1/1, DMC2/1
  BinarySwitch26/1 -> HardwareInputControl2/1
  HardwareInputControl2/1 -> Data Store Write6/1
  HardwareInputControl1/1 -> Data Store Write6/2
  BinarySwitch25/1 -> HardwareInputControl1/1
  Bus Selector3/2 -> Bus Selector8/1  "<CouplerAudio>"
  Bus Selector1/1 -> Vector Concatenate/1  "<MechanicalCouplerState>"
  Bus Selector8/1 -> Vector Concatenate/2  "<MechanicalUncouple>"
  Vector Concatenate/1 -> Display21/1
  Vector Concatenate1/1 -> Display3/1
  Bus Selector10/1 -> Vector Concatenate1/2  "<MechanicalUncouple>"
  Bus Selector9/1 -> Vector Concatenate1/1  "<MechanicalCouplerState>"
  Bus Selector/2 -> Bus Selector10/1  "<CouplerAudio>"
  Selector1/1 -> Bus Selector9/1
  Bus Selector/1 -> Bus Selector13/1  "<Couplers>"
  BinarySwitch9/1 -> Data Type Conversion10/1
  Data Type Conversion10/1 -> Data Store Write3/9
  Data Type Conversion9/1 -> Data Store Write3/10
  BinarySwitch8/1 -> Data Type Conversion9/1
  BinarySwitch7/1 -> Data Type Conversion7/1
  Data Type Conversion7/1 -> Data Store Write3/7
  Data Type Conversion6/1 -> Data Store Write3/8
  BinarySwitch6/1 -> Data Type Conversion6/1
  Bus Selector2/1 -> Selector2/1  "<Coupler>"
  Bus Selector11/1 -> Selector4/1  "<Coupler>"
  Bus Selector12/1 -> Selector3/1  "<Coupler>"
  Bus Selector13/1 -> Selector1/1  "<Coupler>"
